simulink model "atrias_original"  (R2017a)
settings: Solver=ode45  StartTime=0.0  StopTime=sim_t  RelTol=1e-6  EnableMultiTasking=on
values from neighbouring files (symbols this model uses):
  N = grid_slice*1000    [createGrid.m]
  nm = fn_set_vnmc_params(sm, sample_time)    [kernel_scores_NM_mismatch.m]    (also in main_ATRIAS_cluster.m)
  nmc_BLCtrlPar = nmc.BLCtrlPar    [kernel_scores_NM_mismatch.m]    (also in main_ATRIAS_cluster.m)
  nmc_FPCtrlPar = nmc.FPCtrlPar    [kernel_scores_NM_mismatch.m]    (also in main_ATRIAS_cluster.m)
  nmc_LLCtrlPar = nmc.LLCtrlPar    [kernel_scores_NM_mismatch.m]    (also in main_ATRIAS_cluster.m)
  nmc_StCtrlPar = nmc.StCtrlPar    [kernel_scores_NM_mismatch.m]    (also in main_ATRIAS_cluster.m)
  nmc_SwCtrlPar = nmc.SwCtrlPar    [kernel_scores_NM_mismatch.m]    (also in main_ATRIAS_cluster.m)
  nmc_TrCtrlPar = nmc.TrCtrlPar    [kernel_scores_NM_mismatch.m]    (also in main_ATRIAS_cluster.m)
  nStep_switchCtrl = 10    [main_ATRIAS_cluster.m]
  nStep_thr = 1000    [createSimInitial.m]    (also in main_ATRIAS_cluster.m)
  rc_CtrlPar = [rc.k_placement, rc.T_step, rc.Cd, rc.kpt, rc.kdt, rc.desired_theta, rc.desired_z, rc.kpz, rc.kdz]    [kernel_scores_NM_mismatch.m]    (also in main_ATRIAS_cluster.m)
  sm = fn_set_MechParams(sm)    [kernel_scores_NM_mismatch.m]    (also in main_ATRIAS_cluster.m = fn_set_MechParams(sm,perturb))
  test_VNMC = 1    [createSimInitial.m]    (also in main_ATRIAS_cluster.m = 0)
undefined symbols (not defined in the file or in its folder): delta_phi_max, delta_phi_max_buffer, delta_phi_min, DiscIntNeverNeededParam, Discrete, idc, initial_dx_estimate, initial_dy_estimate, initial_dz_estimate, initial_z_estimate, kd_shin_max, kd_shin_min, kd_splay_max, kd_splay_min, kd_thigh_max, kd_thigh_min, kp_shin_max, kp_shin_min, kp_splay_max, kp_splay_min, kp_thigh_max, kp_thigh_min, mc, min_splay_angle, min_splay_buffer, phi_shin_max, phi_shin_max_buffer, phi_shin_min, phi_shin_min_buffer, phi_thigh_max, phi_thigh_max_buffer, phi_thigh_min, phi_thigh_min_buffer, rad, rc, s, sample_time, sgn, sim_d, t_friction, Time, X, Y, Z
libraries: sm_lib x202, nesl_utility x122, simulink x77, simulink_extras x24, fl_lib x16, mblibv1 x4, ctrlSharedLib x4, commnoisgen2 x1, dspswit3 x1
(part 1 of 17)
settings Model: TunableVars=nmc_BLCtrlPar,nmc_FPCtrlPar,nmc_LLCtrlPar,nmc_StCtrlPar,nmc_SwCtrlPar,nmc_TrCtrlPar  TunableVarsStorageClass=Auto,Auto,Auto,Auto,Auto,Auto  TunableVarsTypeQualifier=,,,,,  Creator=smsong  LastModifiedBy=arai
settings DataIOCC: InitialState=SimInitial  LimitDataPoints=on  SaveFinalState=on  SaveCompleteFinalSimState=on  SaveFormat=Array
settings OptimizationCC: EfficientMapNaN2IntZero=off  LifeSpan=inf
settings DebuggingCC: SFUnexpectedBacktrackingDiag=warning  SFNoUnconditionalDefaultTransitionDiag=warning  SFExecutionAtInitializationDiag=none
settings HardwareCC: ProdBitPerPointer=32  ProdBitPerSizeT=32  ProdBitPerPtrDiffT=32  ProdLargestAtomicFloat=None  ProdIntDivRoundTo=Undefined  ProdEndianess=Unspecified  ProdWordSize=32  ProdHWDeviceType=32-bit Generic  TargetBitPerLong=64  TargetBitPerPointer=64  TargetBitPerSizeT=64  TargetBitPerPtrDiffT=64  TargetLongLongMode=on  TargetIntDivRoundTo=Zero  TargetEndianess=LittleEndian  TargetWordSize=64  TargetHWDeviceType=MATLAB Host  ProdEqTarget=off
settings ModelReferenceCC: PropagateSignalLabelsOutOfModel=off
settings CodeAppCC: MaxIdLength=128
settings GRTTargetCC: TargetLangStandard=C89/C90 (ANSI)  CombineOutputUpdateFcns=off  GRTInterface=on  UseToolchainInfoCompliant=off
settings ConfigComp: CovMetricSettings=dw  CovHtmlReporting=on  CovSaveCumulativeToWorkspaceVar=on  CovSaveSingleToWorkspaceVar=on  CovExternalEMLEnable=off
settings ConfigurationSet: Description=SimMechanics 2G
settings ExplorerConfigSet: InternalSimMechanicsExplorerSettings="<ExplorerConfiguration><canonicalview>default</canonicalview><AnimationSetting><BasePlaybackSpeed>1.0</BasePlaybackSpeed><PlaybackSpeedFactor>1.0</PlaybackSpeedFactor></AnimationSetting><TilePanel><TileInfo><Tiles Columns=\"1\" Count=\"1\" Rows=\"1\"><Column Left=\"2\" Weight=\"1\"/><Column Left=\"738\"/><Row Top=\"2\" Weight=\"1\"/><Row Top=\"586\"/><Tile Height=\"1\" Width=\"1\" X=\"0\" Y=\"0\"/></Tiles></TileInfo><SceneInfo><SceneViewer><BGColor><R>1</R><G>1</G><B>1</B></BGColor><Camera><DoPerspective>off</DoPerspective><Position><X>-1.70399005576821305</X><Y>-4.20466739695413683</Y><Z>2.0578773047124157</Z></Position><Center><X>-0.00120101730655930439</X><Y>-0.00299649565581994182</Y><Z>1.48292546750794929</Z></Center><Up><X>0.0468067459368392558</X><Y>0.116782400880656612</Y><Z>0.992053929672855328</Z></Up><ViewLimDist>1</ViewLimDist><YLim>2.524026181051787</YLim><XLim>3.1912470149993899</XLim></Camera></SceneViewer></SceneInfo></TilePanel><MechEditorPanel><Cameras/><GfxPanelCameraMap/><VideoCreator><PlaybackSpeedRatio>1.0</PlaybackSpeedRatio><FrameRate>30</FrameRate><VideoFormat>Motion JPEG AVI</VideoFormat><FrameSize>auto</FrameSize></VideoCreator></MechEditorPanel></ExplorerConfiguration>"

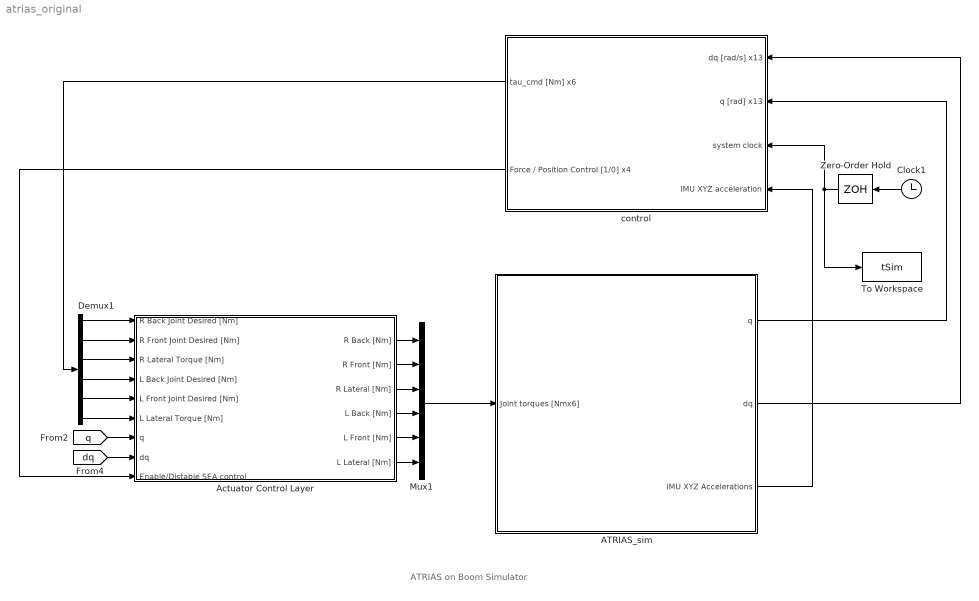
== system atrias_original ==
  note: ATRIAS on Boom Simulator
  ATRIAS_sim : Subsystem
  Actuator Control Layer : Subsystem
  Clock1 : Clock
  Demux1 : Demux  Outputs=6
  Mux1 : Mux  Inputs=6
  To Workspace : ToWorkspace  VariableName=tSim  SaveFormat=Timeseries  SampleTime=-1
      settings: MaxDataPoints=1
  Zero-Order Hold : ZeroOrderHold  SampleTime=sample_time
  control : Subsystem
  wires:
  Clock1/1 -> Zero-Order Hold/1
  Zero-Order Hold/1 -> To Workspace/1, control/3(system clock)
  [q] -> Actuator Control Layer/7(q)
  [dq] -> Actuator Control Layer/8(dq)
  Demux1/1 -> Actuator Control Layer/1(R Back Joint Desired [Nm])
  Demux1/2 -> Actuator Control Layer/2(R Front Joint Desired [Nm])
  Demux1/4 -> Actuator Control Layer/4(L Back Joint Desired [Nm])
  Demux1/5 -> Actuator Control Layer/5(L Front Joint Desired [Nm])
  Demux1/3 -> Actuator Control Layer/3(R Lateral Torque [Nm])
  Demux1/6 -> Actuator Control Layer/6(L Lateral Torque [Nm])
  Actuator Control Layer/3(R Lateral [Nm]) -> Mux1/3
  Actuator Control Layer/1(R Back [Nm]) -> Mux1/1
  Actuator Control Layer/2(R Front [Nm]) -> Mux1/2
  Actuator Control Layer/4(L Back [Nm]) -> Mux1/4
  Actuator Control Layer/5(L Front [Nm]) -> Mux1/5
  Actuator Control Layer/6(L Lateral [Nm]) -> Mux1/6
  Mux1/1 -> ATRIAS_sim/1(Joint torques [Nmx6])
  control/1(tau_cmd [Nm] x6) -> Demux1/1
  control/2(Force / Position Control [1/0] x4) -> Actuator Control Layer/9(Enable/Distable SEA control)
  ATRIAS_sim/2(dq) -> control/1(dq [rad/s] x13)
  ATRIAS_sim/1(q) -> control/2(q [rad] x13)
  ATRIAS_sim/3(IMU XYZ Accelerations) -> control/4(IMU XYZ acceleration)

== system atrias_original/ATRIAS_sim ==
  Joint torques [Nmx6] : Inport
  Acceleration Measurement : Scope  NumInputPorts=3
  Delay : Delay  DelayLength=1  SampleTime=sample_time
  Demux : Demux  Outputs=6
  Demux2 : Demux  Outputs=3
  Discrete Derivative : Subsystem
  Discretize : ZeroOrderHold  SampleTime=sample_time
  Discretize1 : ZeroOrderHold  SampleTime=sample_time
  Discretize2 : ZeroOrderHold  SampleTime=sample_time
  Gaussian Noise Generator : commnoisgen2/Gaussian Noise Generator  m=0  d=sm.sensor_noise_variance  s=41  Ts=sample_time  frameBased=off  sampPerFrame=1  orient=off  outDataType=double
  Mechanical System Layer : Subsystem
  Mux : Mux  Inputs=13
  Sum : Sum  Inputs=|++
  q : Outport  InitialOutput=[0]
  dq : Outport  Port=2  InitialOutput=[0]
  IMU XYZ Accelerations : Outport  Port=3  InitialOutput=[0]
  wires:
  Mechanical System Layer/1(R Back Joint [rad]) -> Mux/1
  Mechanical System Layer/2(R Back Gear [rad]) -> Mux/2
  Mechanical System Layer/3(R Front Joint [rad]) -> Mux/3
  Mechanical System Layer/4(R Front Gear [rad]) -> Mux/4
  Mechanical System Layer/5(L Back Joint [rad]) -> Mux/5
  Mechanical System Layer/6(L Back Gear [rad]) -> Mux/6
  Mechanical System Layer/7(L Front Joint [rad]) -> Mux/7
  Mechanical System Layer/8(L Front Gear [rad]) -> Mux/8
  Mechanical System Layer/9(R Lateral [rad]) -> Mux/9
  Mechanical System Layer/10(L Lateral [rad]) -> Mux/10
  Mechanical System Layer/11(Torso Roll [rad]) -> Mux/11
  Mechanical System Layer/12(Torso Yaw [rad]) -> Mux/12
  Mechanical System Layer/13(Torso Pitch [rad]) -> Mux/13
  Demux/1 -> Mechanical System Layer/1(R Back Motor [Nm])
  Demux/2 -> Mechanical System Layer/2(R Front Motor [Nm])
  Demux/3 -> Mechanical System Layer/3(R Lat Motor [Nm])
  Demux/4 -> Mechanical System Layer/4(L Back Motor [Nm])
  Demux/5 -> Mechanical System Layer/5(L Front Motor [Nm])
  Demux/6 -> Mechanical System Layer/6(L Lat Motor [Nm])
  Discretize/1 -> Sum/1
  Gaussian Noise Generator/1 -> ?
  Delay/1 -> Demux/1
  Mux/1 -> Discretize/1
  Mechanical System Layer/14("IMU XYZ Acclerations [m/s^2] x3 ") -> Discretize1/1
  Sum/1 -> q/1, Discrete Derivative/1(q)
  Joint torques [Nmx6]/1 -> Delay/1
  Discrete Derivative/1(dq) -> dq/1
  Demux2/3 -> Acceleration Measurement/3
  Demux2/1 -> Acceleration Measurement/1
  Demux2/2 -> Acceleration Measurement/2
  Discretize1/1 -> Demux2/1, Discretize2/1
  Discretize2/1 -> IMU XYZ Accelerations/1

== system atrias_original/Actuator Control Layer ==
  note: ATRIAS Actuation Control Layer
  note: q Order:
      |
      | backJointR
      | backGearR
      | frontJointR
      | frontGearR
      |
      | backJointL
      | backGearL
      | frontJointL
      | frontGearL
      |
      | latR
      | latL
      |
      | boomRoll
      | boomYaw
      | boomPitch
  R Back Joint Desired [Nm] : Inport
  R Front Joint Desired [Nm] : Inport  Port=2
  R Lateral Torque [Nm] : Inport  Port=3
  L Back Joint Desired [Nm] : Inport  Port=4
  L Front Joint Desired [Nm] : Inport  Port=5
  L Lateral Torque [Nm] : Inport  Port=6
  q : Inport  Port=7
  dq : Inport  Port=8
  Enable/Distable SEA control : Inport  Port=9
  Demux : Demux
  Gain : Gain  Gain=1/sm.mu_hmotor
  Gain1 : Gain  Gain=1/sm.mu_hmotor
  Mux : Mux
  Mux{3,5..7} (4 alike) : Mux  Inputs=2
  Product : Product
  "RB, RF, LB, LF" : Scope  NumInputPorts=4
  SEA Controller (Torque) : Subsystem
  Selector1 : Selector  InputPortWidth=13  IndexOptions=Index vector (dialog)  Indices=[2 4 6 8]  OutputSizes=1
  Selector10 : Selector  InputPortWidth=4  IndexOptions=Index vector (dialog)  Indices=[4]  OutputSizes=1
  Selector11 : Selector  InputPortWidth=4  IndexOptions=Index vector (dialog)  Indices=[2]  OutputSizes=1
  Selector12 : Selector  InputPortWidth=4  IndexOptions=Index vector (dialog)  Indices=[2]  OutputSizes=1
  Selector13 : Selector  InputPortWidth=4  IndexOptions=Index vector (dialog)  Indices=[1]  OutputSizes=1
  Selector14 : Selector  InputPortWidth=4  IndexOptions=Index vector (dialog)  Indices=[1]  OutputSizes=1
  Selector15 : Selector  InputPortWidth=13  IndexOptions=Index vector (dialog)  Indices=[1 3 5 7]  OutputSizes=1
  Selector16 : Selector  InputPortWidth=13  IndexOptions=Index vector (dialog)  Indices=[1 3 5 7]  OutputSizes=1
  Selector2 : Selector  InputPortWidth=13  IndexOptions=Index vector (dialog)  Indices=[2 4 6 8]  OutputSizes=1
  Selector7 : Selector  InputPortWidth=4  IndexOptions=Index vector (dialog)  Indices=[3]  OutputSizes=1
  Selector8 : Selector  InputPortWidth=4  IndexOptions=Index vector (dialog)  Indices=[3]  OutputSizes=1
  Selector9 : Selector  InputPortWidth=4  IndexOptions=Index vector (dialog)  Indices=[4]  OutputSizes=1
  Toggle SEA control : Subsystem
  tau_cmd [Nm] : Scope
  torque_command : ToWorkspace  VariableName=tau_cmd1  SampleTime=-1
  R Back [Nm] : Outport  InitialOutput=[0]
  R Front [Nm] : Outport  Port=2  InitialOutput=[0]
  R Lateral [Nm] : Outport  Port=3  InitialOutput=[0]
  L Back [Nm] : Outport  Port=4  InitialOutput=[0]
  L Front [Nm] : Outport  Port=5  InitialOutput=[0]
  L Lateral [Nm] : Outport  Port=6  InitialOutput=[0]
  wires:
  L Lateral Torque [Nm]/1 -> Gain1/1
  R Lateral Torque [Nm]/1 -> Gain/1
  Enable/Distable SEA control/1 -> SEA Controller (Torque)/6(Enable/Disable [1/0] x4), Product/2, Toggle SEA control/3(SEA Control on or off [1/0] x4)
  SEA Controller (Torque)/2(tau_cmd sagittal [Nm] x4) -> torque_command/1, Toggle SEA control/1(SEA Control Torques [Nm] x4)
  Product/1 -> Selector13/1, Selector9/1, Selector7/1, Selector11/1
  Demux/3 -> L Back [Nm]/1
  Demux/4 -> L Front [Nm]/1
  R Back Joint Desired [Nm]/1 -> Mux/1
  R Front Joint Desired [Nm]/1 -> Mux/2
  L Back Joint Desired [Nm]/1 -> Mux/3
  L Front Joint Desired [Nm]/1 -> Mux/4
  Selector15/1 -> SEA Controller (Torque)/2(phi_load [rad] x4)
  Selector2/1 -> SEA Controller (Torque)/3(phi_gear [rad] x4)
  Selector1/1 -> SEA Controller (Torque)/5(dphi_gear [rad/s] x4)
  Mux3/1 -> "RB, RF, LB, LF"/3
  Selector7/1 -> Mux3/1
  Selector8/1 -> Mux3/2
  Mux5/1 -> "RB, RF, LB, LF"/4
  Selector9/1 -> Mux5/1
  Selector10/1 -> Mux5/2
  Mux6/1 -> "RB, RF, LB, LF"/2
  Selector11/1 -> Mux6/1
  Selector12/1 -> Mux6/2
  Mux7/1 -> "RB, RF, LB, LF"/1
  SEA Controller (Torque)/1(tau_measured sagittal [Nm] x4) -> Selector14/1, Selector12/1, Selector8/1, Selector10/1
  Selector14/1 -> Mux7/2
  [dq] -> Selector16/1, Selector1/1
  Selector16/1 -> SEA Controller (Torque)/4(dphi_load [rad/s] x4)
  [q] -> Selector2/1, Selector15/1
  q/1 -> [q]
  dq/1 -> [dq]
  Demux/2 -> R Front [Nm]/1
  Demux/1 -> R Back [Nm]/1
  Selector13/1 -> Mux7/1
  Toggle SEA control/1(Motor Torque Commands [Nm] x4) -> tau_cmd [Nm]/1, Demux/1
  Mux/1 -> SEA Controller (Torque)/1(tau_des sagittal [Nm] x4), Toggle SEA control/2(Non-SEA control Torques [Nm] x4), Product/1
  Gain/1 -> R Lateral [Nm]/1
  Gain1/1 -> L Lateral [Nm]/1

== system atrias_original/control ==
  note: Robot-NMM Interface
  note: Neuromuscular Model
  note: Data
  note: Raibert Control
  note: Switch
  dq [rad/s] x13 : Inport
  q [rad] x13 : Inport  Port=2
  system clock : Inport  Port=3
  IMU XYZ acceleration : Inport  Port=4
  Data : Subsystem
  Demux3 : Demux
  Demux4 : Demux  Outputs=6
  Mux{,1,3..4} (4 alike) : Mux  Inputs=2
  Mux2 : Mux  Inputs=6
  Mux7 : Mux
  Mux8 : Mux
  NMM vs Raibert : Scope  NumInputPorts=4
  RC control : Subsystem
  Robot-to-NMM Interface : Subsystem
  Virtual Neuromuscular Control : Subsystem  SystemSampleTime=sample_time
  switch Ctrl : Subsystem
  tau_cmd [Nm] x6 : Outport
  Force / Position Control [1/0] x4 : Outport  Port=2  OutputWhenDisabled=reset  InitialOutput=[0 0 0 0 0 0]
  tag scope: LFootCnt=global, LLLoad=global, LLat_ctrl_trq=global, LLength=global, Lalpha=global, LdLength=global, Ldalpha=global, Ldgamma=global, Lgamma=global, Lphi12=global, Lphi23=global, Lshin_ctrl_trq=global, Lshin_ctrl_trq_NMM=global, Lshin_ctrl_trq_VMC=global, LtauB=global, LtauF=global, Lthigh_ctrl_trq=global, Lthigh_ctrl_trq_NMM=global, Lthigh_ctrl_trq_VMC=global, RFootCnt=global, RLLoad=global, RLat_ctrl_trq=global, RLength=global, Ralpha=global, RdLength=global, Rdalpha=global, Rdgamma=global, Rgamma=global, Rphi12=global, Rphi23=global, Rshin_ctrl_trq=global, Rshin_ctrl_trq_NMM=global, Rshin_ctrl_trq_VMC=global, RtauB=global, RtauF=global, Rthigh_ctrl_trq=global, Rthigh_ctrl_trq_NMM=global, Rthigh_ctrl_trq_VMC=global, dq=global, k_L=global, k_R=global, q=global
  wires:
  [Rshin_ctrl_trq] -> Mux2/1
  [Rthigh_ctrl_trq] -> Mux2/2
  [RLat_ctrl_trq] -> Mux2/3
  [Lshin_ctrl_trq] -> Mux2/4
  [Lthigh_ctrl_trq] -> Mux2/5
  [LLat_ctrl_trq] -> Mux2/6
  dq [rad/s] x13/1 -> [dq]
  q [rad] x13/1 -> [q]
  [q] -> Robot-to-NMM Interface/1(q_discrete [rad] x13)
  [dq] -> Robot-to-NMM Interface/2(dq_discrete [rad/2] x13)
  Robot-to-NMM Interface/23(L Leg Load [bw]) -> [LLLoad]
  Robot-to-NMM Interface/24(R Leg Load [bw]) -> [RLLoad]
  Robot-to-NMM Interface/6(L Alpha [rad]) -> [Lalpha]
  Robot-to-NMM Interface/5(R Alpha [rad]) -> [Ralpha]
  Robot-to-NMM Interface/8(L Leg Length [m]) -> [LLength]
  Robot-to-NMM Interface/7(R Leg Length [m]) -> [RLength]
  Robot-to-NMM Interface/4(L_tau_front_meas [Nm]) -> [LtauF]
  Robot-to-NMM Interface/3(L_tau_back_meas [Nm]) -> [LtauB]
  Robot-to-NMM Interface/2(R_tau_front_meas [Nm]) -> [RtauF]
  Robot-to-NMM Interface/1(R_tau_back_meas [Nm]) -> [RtauB]
  Robot-to-NMM Interface/11(R virtual knee angle [rad]) -> [Rphi12]
  Robot-to-NMM Interface/12(R virtual hip angle [rad]) -> [Rphi23]
  Robot-to-NMM Interface/13(L virtual knee angle [rad]) -> [Lphi12]
  Robot-to-NMM Interface/14(L virtual hip angle [rad]) -> [Lphi23]
  Robot-to-NMM Interface/16(L Jacobian Constant (k)) -> [k_L]
  Robot-to-NMM Interface/15(R Jacobian Constant (k)) -> [k_R]
  Robot-to-NMM Interface/21(R dAlpha [rad/s]) -> [Rdalpha]
  Robot-to-NMM Interface/22(L dAlpha [rad/s]) -> [Ldalpha]
  Robot-to-NMM Interface/17(Rgamma [rad]) -> [Rgamma]
  Robot-to-NMM Interface/18(Lgamma [rad]) -> [Lgamma]
  Robot-to-NMM Interface/19(Rdgamma [rad]) -> [Rdgamma]
  Robot-to-NMM Interface/20(Ldgamma [rad]) -> [Ldgamma]
  Robot-to-NMM Interface/10(R Leg Length Velocity [m/s]) -> [RdLength]
  Robot-to-NMM Interface/9(L Leg Length Velocity [m/s]) -> [LdLength]
  Demux4/1 -> [Rshin_ctrl_trq_VMC]
  Demux4/2 -> [Rthigh_ctrl_trq_VMC]
  Demux4/3 -> [RLat_ctrl_trq]
  Demux4/4 -> [Lshin_ctrl_trq_VMC]
  Virtual Neuromuscular Control/1(RtauB_des [Nm]) -> [Rshin_ctrl_trq_NMM]
  Virtual Neuromuscular Control/2(RtauF_des [Nm]) -> [Rthigh_ctrl_trq_NMM]
  Virtual Neuromuscular Control/3(LtauB_des [Nm]) -> [Lshin_ctrl_trq_NMM]
  Virtual Neuromuscular Control/4(LtauF_des [Nm]) -> [Lthigh_ctrl_trq_NMM]
  [Rshin_ctrl_trq_NMM] -> Mux/1, Mux7/1
  [Rthigh_ctrl_trq_NMM] -> Mux1/1, Mux7/2
  [Lshin_ctrl_trq_NMM] -> Mux3/1, Mux7/3
  [Lthigh_ctrl_trq_NMM] -> Mux4/1, Mux7/4
  [Rshin_ctrl_trq_VMC] -> Mux/2, Mux8/1
  [Rthigh_ctrl_trq_VMC] -> Mux1/2, Mux8/2
  [Lshin_ctrl_trq_VMC] -> Mux3/2, Mux8/3
  [Lthigh_ctrl_trq_VMC] -> Mux4/2, Mux8/4
  Demux3/4 -> [Lthigh_ctrl_trq]
  Demux3/3 -> [Lshin_ctrl_trq]
  Demux3/2 -> [Rthigh_ctrl_trq]
  Demux3/1 -> [Rshin_ctrl_trq]
  Robot-to-NMM Interface/26(L Contact [0/1]) -> [LFootCnt]
  Robot-to-NMM Interface/25(R Contact [0/1]) -> [RFootCnt]
  [dq] -> RC control/2(dq_cmu)
  [q] -> RC control/1(q_cmu)
  system clock/1 -> RC control/3(system clock)
  RC control/2(Motor Torque Command [Nm] x6) -> Demux4/1
  Demux4/5 -> [Lthigh_ctrl_trq_VMC]
  Demux4/6 -> [LLat_ctrl_trq]
  RC control/1(Force / Position Control [1/0] x4) -> Force / Position Control [1/0] x4/1
  Robot-to-NMM Interface/27(Entering stance) -> RC control/4(Entering Stance)
  IMU XYZ acceleration/1 -> RC control/5(Body XYZ Acceleration [m/s^2] x3)
  Mux/1 -> NMM vs Raibert/1
  Mux1/1 -> NMM vs Raibert/2
  Mux3/1 -> NMM vs Raibert/3
  Mux4/1 -> NMM vs Raibert/4
  switch Ctrl/1(selected) -> Demux3/1
  Mux7/1 -> switch Ctrl/1(VNMC)
  Mux8/1 -> switch Ctrl/2(RC)
  Mux2/1 -> tau_cmd [Nm] x6/1

== system atrias_original/ATRIAS_sim/Discrete Derivative ==
  q : Inport
  Gain1 : Gain  Gain=1/sample_time
  discrete difference : Subsystem
  dq : Outport
  wires:
  q/1 -> discrete difference/1(in)
  Gain1/1 -> dq/1
  discrete difference/1(out) -> Gain1/1

== system atrias_original/ATRIAS_sim/Mechanical System Layer ==
  R Back Motor [Nm] : Inport
  R Front Motor [Nm] : Inport  Port=2
  R Lat Motor [Nm] : Inport  Port=3
  L Back Motor [Nm] : Inport  Port=4
  L Front Motor [Nm] : Inport  Port=5
  L Lat Motor [Nm] : Inport  Port=6
  Boom : Subsystem
      mask Display: image('../images/boom.png');
  Boom Base : Subsystem
      mask Display: image('../images/boom_base.png');
  Demux : Demux  Outputs=3
  Demux1 : Demux  Outputs=3
  Demux2 : Demux  Outputs=3
  Floor : Subsystem
  Floor Frame : sm_lib/Frames and Transforms/Rigid Transform  TranslationMethod=Cartesian  TranslationStandardOffset=0  TranslationLengthUnit=m  TranslationStandardAxis=+Z  TranslationCartesianOffset=[0 -0.03 0]  TranslationROffset=0  TranslationROffsetUnits=m  TranslationZOffset=0  TranslationZOffsetUnits=m  TranslationThetaOffset=0  TranslationThetaOffsetUnits=deg  RotationMethod=AlignedAxes  RotationAngleUnits=deg  RotationStandardAxis=+Z  RotationAngle=0  RotationArbitraryAxis=[0 0 1]  FollAlignAxisA=+Z  BaseAlignAxisA=+Y  FollAlignAxisB=+X  BaseAlignAxisB=+X  RotationSequenceAxes=FollowerAxes  RotationSequence=XYX  RotationSequenceAngles=[0 0 0]  RotationSequenceAnglesUnits=deg  RotationMatrix=[1 0 0; 0 1 0; 0 0 1]
  From1 : From  Commented=on  GotoTag=GlobalRightLeftPrimary  TagVisibility=global
  From55 : From  Commented=on  GotoTag=RightLeftPrimary
  Gain : Gain  Commented=on  Gain=[1 -1 1]
  Goto : Goto  Commented=on  GotoTag=GlobalPrimaryGRF  TagVisibility=global
  Ground : Subsystem
  Ground Height : Scope  Commented=on
  L GRF : Scope
  L Ground Contact : Subsystem  SystemSampleTime=t_friction
  L Hip Shaft : Subsystem
      mask Display: image(flipdim(imread('../images/hipshaft.JPG'),2));
  L Leg : Subsystem
      mask Display: image('../images/leg.JPG');
  Left Hip Roll Joint : Subsystem
  Pitch Joint : Subsystem
  R GRF : Scope
  R Ground Contact : Subsystem  SystemSampleTime=t_friction
  R Hip Shaft : Subsystem
      mask Display: image('../images/hipshaft.JPG');
  R Leg : Subsystem
      mask Display: image('../images/leg.JPG');
  Right Hip Roll Joint : Subsystem
  Selector : Selector  Commented=on  InputPortWidth=3  IndexOptions=Index vector (dialog)  Indices=[1 3 2]  OutputSizes=1
  Sum : Sum  Inputs=2
  Switch : Switch  Commented=on  Criteria=u2 ~= 0
  Switch1 : Switch  Commented=on  Criteria=u2 ~= 0
  Terminator : Terminator
  Terminator1 : Terminator
  Terminator2 : Terminator
  Torso : Subsystem
      mask Display: image('../images/torso.png');
  Winch : Subsystem
  World to Yup : sm_lib/Frames and Transforms/Rigid Transform  TranslationMethod=None  TranslationStandardOffset=0  TranslationLengthUnit=m  TranslationStandardAxis=+Z  TranslationCartesianOffset=0  TranslationROffset=0  TranslationROffsetUnits=m  TranslationZOffset=0  TranslationZOffsetUnits=m  TranslationThetaOffset=0  TranslationThetaOffsetUnits=deg  RotationMethod=AlignedAxes  RotationAngleUnits=deg  RotationStandardAxis=+Z  RotationAngle=0  RotationArbitraryAxis=[0 0 1]  FollAlignAxisA=+Y  BaseAlignAxisA=+Z  FollAlignAxisB=+X  BaseAlignAxisB=+X  RotationSequenceAxes=FollowerAxes  RotationSequence=XYX  RotationSequenceAngles=[0 0 0]  RotationSequenceAnglesUnits=deg  RotationMatrix=[1 0 0; 0 1 0; 0 0 1]
  Yaw Joint : Subsystem
  Yaw Shaft : Subsystem
      mask Display: image('../images/boom_yaw_shaft.png');
  R Back Joint [rad] : Outport
  R Back Gear [rad] : Outport  Port=2
  R Front Joint [rad] : Outport  Port=3
  R Front Gear [rad] : Outport  Port=4
  L Back Joint [rad] : Outport  Port=5
  L Back Gear [rad] : Outport  Port=6
  L Front Joint [rad] : Outport  Port=7
  L Front Gear [rad] : Outport  Port=8
  R Lateral [rad] : Outport  Port=9
  L Lateral [rad] : Outport  Port=10
  Torso Roll [rad] : Outport  Port=11
  Torso Yaw [rad] : Outport  Port=12
  Torso Pitch [rad] : Outport  Port=13
  "IMU XYZ Acclerations [m/s^2] x3 " : Outport  Port=14
  tag scope: GRFz=global
  wires:
  L Leg/1(Shin Joint [rad]) -> L Back Joint [rad]/1
  R Back Motor [Nm]/1 -> R Leg/1(Shin Motor [Nm])
  L Back Motor [Nm]/1 -> L Leg/1(Shin Motor [Nm])
  Right Hip Roll Joint/1(Hip Roll [rad]) -> R Lateral [rad]/1
  L Leg/3(Thigh Joint [rad]) -> L Front Joint [rad]/1
  Left Hip Roll Joint/1(Hip Roll [rad]) -> L Lateral [rad]/1
  L Leg/4(Thigh Gear [rad]) -> L Front Gear [rad]/1
  R Leg/1(Shin Joint [rad]) -> R Back Joint [rad]/1
  R Leg/2(Shin Gear [rad]) -> R Back Gear [rad]/1
  L Leg/2(Shin Gear [rad]) -> L Back Gear [rad]/1
  R Leg/4(Thigh Gear [rad]) -> R Front Gear [rad]/1
  L Front Motor [Nm]/1 -> L Leg/2("Thigh Motor [Nm]  ")
  R Lat Motor [Nm]/1 -> Right Hip Roll Joint/1(Hip Motor [Nm])
  R Front Motor [Nm]/1 -> R Leg/2("Thigh Motor [Nm]  ")
  L Lat Motor [Nm]/1 -> Left Hip Roll Joint/1(Hip Motor [Nm])
  R Leg/3(Thigh Joint [rad]) -> R Front Joint [rad]/1
  Pitch Joint/1(Pitch [rad]) -> Terminator/1
  Yaw Joint/1(Yaw [rad]) -> Terminator1/1
  From55/1 -> Switch/2
  Switch/1 -> Ground Height/1
  L Ground Contact/2(zGround) -> Switch/3
  R Ground Contact/2(zGround) -> Switch/1
  Torso/1(IMU XYZ Accelerations [m/s^2] x3) -> "IMU XYZ Acclerations [m/s^2] x3 "/1
  Torso/2(IMU Orientation [rad x3]) -> Demux/1
  Demux/1 -> Torso Roll [rad]/1
  Demux/2 -> Torso Pitch [rad]/1
  Winch/1(Boom Roll [rad]) -> Terminator2/1
  Demux/3 -> Torso Yaw [rad]/1
  From1/1 -> Switch1/2
  L Ground Contact/1(GRF) -> Demux1/1, Switch1/3, L GRF/1
  R Ground Contact/1(GRF) -> Demux2/1, Switch1/1, R GRF/1
  Switch1/1 -> Selector/1
  Selector/1 -> Gain/1
  Gain/1 -> Goto/1
  Demux1/3 -> Sum/1
  Demux2/3 -> Sum/2
  Sum/1 -> [GRFz]
  connections:
  Torso/LConn1 -- Left Hip Roll Joint/RConn1
  Right Hip Roll Joint/RConn1 -- R Hip Shaft/RConn1
  Winch/RConn2 -- Yaw Shaft/RConn1
  Left Hip Roll Joint/LConn1 -- L Hip Shaft/LConn1
  R Ground Contact/LConn1 -- R Leg/LConn1
  R Leg/RConn1 -- R Hip Shaft/LConn1
  Torso/LConn2 -- Right Hip Roll Joint/LConn1
  L Ground Contact/LConn1 -- L Leg/RConn1
  Pitch Joint/LConn1 -- Torso/RConn1
  Floor Frame/RConn1 -- Floor/LConn1
  World to Yup/LConn1 -- Ground/RConn1
  Boom/LConn1 -- Winch/RConn1
  Yaw Shaft/LConn1 -- Yaw Joint/RConn1
  Yaw Joint/LConn1 -- Boom Base/RConn1
  Pitch Joint/RConn1 -- Boom/RConn1
  L Hip Shaft/RConn1 -- L Leg/LConn1
  Floor Frame/LConn1 -- World to Yup/RConn1 -- Boom Base/LConn1

== system atrias_original/Actuator Control Layer/SEA Controller (Torque) ==
  tau_des sagittal [Nm] x4 : Inport
  phi_load [rad] x4 : Inport  Port=2
  phi_gear [rad] x4 : Inport  Port=3
  dphi_load [rad/s] x4 : Inport  Port=4
  dphi_gear [rad/s] x4 : Inport  Port=5
  Enable/Disable [1/0] x4 : Inport  Port=6
  Desired Torque Derivative : Subsystem
  Detect Change : simulink/Logic and Bit Operations/Detect Change  vinit=0  InputProcessing=Inherited  OutDataTypeStr=boolean
  Spring Stiffness1 : Gain  Gain=mc.k_leg_spring
  Spring Stiffness2 : Gain  Gain=mc.k_leg_spring
  Sum10 : Sum  Inputs=-+|
  Sum11 : Sum  Inputs=|++
  Sum6 : Sum  Inputs=-+|
  Sum7 : Sum  Inputs=|+-
  Sum8 : Sum  Inputs=+++
  Sum9 : Sum  Inputs=|+-
  Torque Limiter (outside) 1 : Saturate  UpperLimit=sm.LEG_MTR_MAX_TORQUE  LowerLimit=-sm.LEG_MTR_MAX_TORQUE  ZeroCross=off
      settings: AttributesFormatString=Hi: %<UpperLimit>\nLo: %<LowerLimit>
  kd_gain : Gain  Description=xPCTag(1)=kd_sea_torque;  Gain=mc.kd_sea_torque
  kd_gain2 : Gain  Description=xPCTag(1)=kd_sea_torque;  Gain=mc.kp_sea_torque
  tau_measured sagittal [Nm] x4 : Outport
  tau_cmd sagittal [Nm] x4 : Outport  Port=2
  wires:
  Sum9/1 -> kd_gain2/1
  Torque Limiter (outside) 1/1 -> tau_cmd sagittal [Nm] x4/1
  kd_gain2/1 -> Sum11/1
  kd_gain/1 -> Sum11/2
  Sum11/1 -> Sum8/2
  Sum6/1 -> Spring Stiffness1/1
  Sum8/1 -> Torque Limiter (outside) 1/1
  Sum7/1 -> kd_gain/1
  dphi_gear [rad/s] x4/1 -> Sum10/2
  dphi_load [rad/s] x4/1 -> Sum10/1
  Spring Stiffness2/1 -> Sum7/2
  Sum10/1 -> Spring Stiffness2/1
  Desired Torque Derivative/1(Derivative x4) -> Sum7/1
  phi_gear [rad] x4/1 -> Sum6/2
  phi_load [rad] x4/1 -> Sum6/1
  Spring Stiffness1/1 -> tau_measured sagittal [Nm] x4/1, Sum9/2, Sum8/1
  Detect Change/1 -> Desired Torque Derivative/2(Reset [1/0] x4)
  tau_des sagittal [Nm] x4/1 -> Desired Torque Derivative/1(Signal x4), Sum9/1
  Enable/Disable [1/0] x4/1 -> Detect Change/1

== system atrias_original/Actuator Control Layer/Toggle SEA control ==
  SEA Control Torques [Nm] x4 : Inport
  Non-SEA control Torques [Nm] x4 : Inport  Port=2
  SEA Control on or off [1/0] x4 : Inport  Port=3
  Demux2 : Demux
  Demux3 : Demux
  Demux4 : Demux
  Mux1 : Mux
  Switch{,1..3} (4 alike) : Switch  Criteria=u2 > Threshold
  Motor Torque Commands [Nm] x4 : Outport
  wires:
  SEA Control Torques [Nm] x4/1 -> Demux4/1
  Demux2/3 -> Switch3/2
  Switch3/1 -> Mux1/3
  Demux4/4 -> Switch2/1
  Demux2/1 -> Switch1/2
  Demux4/3 -> Switch3/1
  Demux3/1 -> Switch1/3
  Demux2/2 -> Switch/2
  Demux3/3 -> Switch3/3
  Demux3/2 -> Switch/3
  Demux3/4 -> Switch2/3
  Switch2/1 -> Mux1/4
  Demux4/1 -> Switch1/1
  SEA Control on or off [1/0] x4/1 -> Demux2/1
  Demux4/2 -> Switch/1
  Non-SEA control Torques [Nm] x4/1 -> Demux3/1
  Demux2/4 -> Switch2/2
  Mux1/1 -> Motor Torque Commands [Nm] x4/1
  Switch/1 -> Mux1/2
  Switch1/1 -> Mux1/1

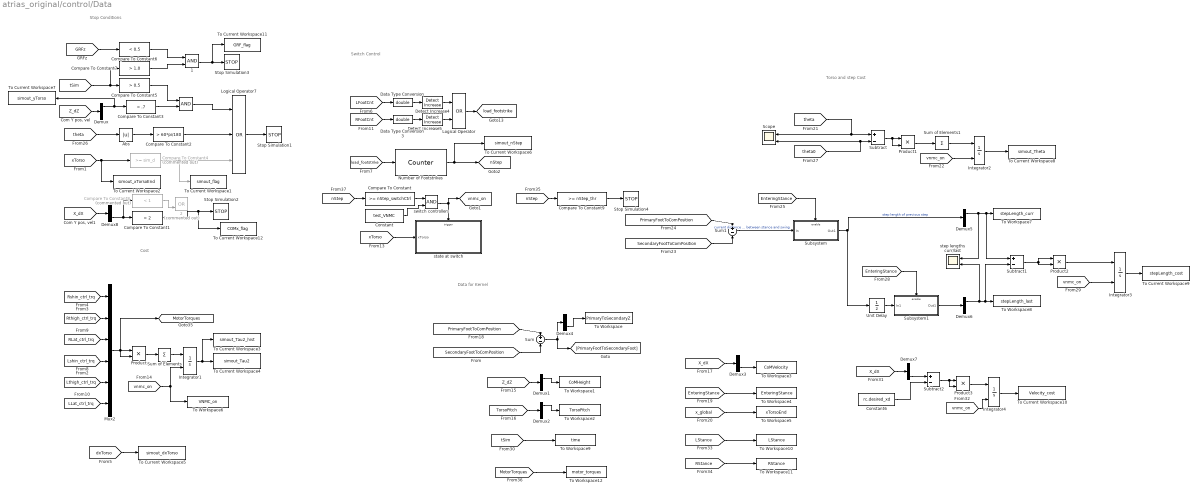
== system atrias_original/control/Data ==
  note: Stop Conditions
  note: Cost
  note: Switch Control
  note: Data for Kernel
  note: Torso and step Cost
  " " : Logic  AllPortsSameDT=off  OutDataTypeStr=boolean
  " 1" : Logic  AllPortsSameDT=off  OutDataTypeStr=boolean
  " 2" : Logic  Commented=on  Operator=OR  AllPortsSameDT=off  OutDataTypeStr=boolean
  Abs : Abs
  Compare To Constant : simulink/Logic and Bit Operations/Compare To Constant  relop=>=  const=nStep_switchCtrl  OutDataTypeStr=boolean
  Compare To Constant1 : simulink/Logic and Bit Operations/Compare To Constant  relop=>  const=2  OutDataTypeStr=boolean
  Compare To Constant2 : simulink/Logic and Bit Operations/Compare To Constant  relop=>  const=60*pi/180  OutDataTypeStr=boolean
  Compare To Constant3 : simulink/Logic and Bit Operations/Compare To Constant  relop=<  const=.7  OutDataTypeStr=boolean
  Compare To Constant4 : simulink/Logic and Bit Operations/Compare To Constant  Commented=on  relop=>=  const=sim_d  OutDataTypeStr=boolean
  Compare To Constant5 : simulink/Logic and Bit Operations/Compare To Constant  relop=>  const=0.5  OutDataTypeStr=boolean
  Compare To Constant6 : simulink/Logic and Bit Operations/Compare To Constant  relop=<  const=0.5  OutDataTypeStr=boolean  ZeroCross=off
  Compare To Constant7 : simulink/Logic and Bit Operations/Compare To Constant  relop=>  const=1.0  OutDataTypeStr=boolean  ZeroCross=off
  Compare To Constant8 : simulink/Logic and Bit Operations/Compare To Constant  Commented=on  relop=<  const=1  OutDataTypeStr=boolean
  Compare To Constant9 : simulink/Logic and Bit Operations/Compare To Constant  relop=>=  const=nStep_thr  OutDataTypeStr=boolean
  Constant : Constant  Value=test_VNMC
  Constant6 : Constant  Value=rc.desired_xd
  Data Type Conversion : DataTypeConversion  OutDataTypeStr=double
  Data Type Conversion3 : DataTypeConversion  OutDataTypeStr=double
  Demux{,1..3,7..8} (6 alike) : Demux  Outputs=2
  Demux4 : Demux  Outputs=3
  Demux5 : Demux  Outputs=3
  Demux6 : Demux  Outputs=3
  Detect Increase4 : simulink/Logic and Bit Operations/Detect Increase  vinit=0.0  InputProcessing=Inherited  OutDataTypeStr=boolean
  Detect Increase5 : simulink/Logic and Bit Operations/Detect Increase  vinit=0.0  InputProcessing=Inherited  OutDataTypeStr=boolean
  Integrator{1..4} (4 alike) : Integrator  ExternalReset=rising  ZeroCross=off
  Logical Operator : Logic  Operator=OR  AllPortsSameDT=off  OutDataTypeStr=boolean
  Logical Operator7 : Logic  Operator=OR  Inputs=3  AllPortsSameDT=off  OutDataTypeStr=boolean
  Mux2 : Mux  Inputs=6
  Number of Footstrikes : dspswit3/Counter  Direction=Up  CountEvent=Rising edge  CounterSize=User defined  MaxCount=255  InitialCount=0  Output=Count  HitValue=4  ResetInput=off  SamplesPerFrame=1  Ts=1  CntDtype=double  HitDtype=Boolean
  Product{,1..3} (4 alike) : Product
  Scope : Scope  NumInputPorts=2
  Stop Simulation{1..4} (4 alike) : Stop
  Subsystem : Subsystem
  Subsystem1 : Subsystem
  Subtract : Sum  Inputs=+-
  Subtract1 : Sum  Inputs=+-
  Subtract2 : Sum  Inputs=+-
  Sum : Sum  Inputs=+-
  Sum of Elements : Sum  Inputs=+
  Sum of Elements1 : Sum  Inputs=+
  Sum1 : Sum  Inputs=+-
  To Current Workspace1 : ToWorkspace  VariableName=simout_flag  SaveFormat=Structure  SampleTime=-1
      settings: MaxDataPoints=1
  To Current Workspace10 : ToWorkspace  VariableName=Velocity_cost  SaveFormat=Structure With Time  SampleTime=-1
  To Current Workspace11 : ToWorkspace  VariableName=GRF_flag  SaveFormat=Structure  SampleTime=-1
      settings: MaxDataPoints=1
  To Current Workspace12 : ToWorkspace  VariableName=COMx_flag  SaveFormat=Structure  SampleTime=-1
      settings: MaxDataPoints=1
  To Current Workspace2 : ToWorkspace  VariableName=simout_xTorsoEnd  SaveFormat=Structure With Time  SampleTime=-1
  To Current Workspace3 : ToWorkspace  VariableName=simout_Tau2_hist  SaveFormat=Structure With Time  SampleTime=-1
  To Current Workspace4 : ToWorkspace  VariableName=simout_Tau2  SaveFormat=Structure  SampleTime=-1
      settings: MaxDataPoints=1
  To Current Workspace5 : ToWorkspace  VariableName=simout_dxTorso  SaveFormat=Structure With Time  SampleTime=-1
  To Current Workspace6 : ToWorkspace  VariableName=simout_nStep  SaveFormat=Structure With Time  SampleTime=-1
  To Current Workspace7 : ToWorkspace  VariableName=simout_yTorso  SaveFormat=Structure With Time  SampleTime=-1
  To Current Workspace8 : ToWorkspace  VariableName=simout_Theta  SaveFormat=Structure With Time  SampleTime=-1
  To Current Workspace9 : ToWorkspace  VariableName=stepLength_cost  SaveFormat=Structure  SampleTime=-1
  To Workspace : ToWorkspace  VariableName=PrimaryToSecondaryZ  SaveFormat=Structure With Time  SampleTime=-1
  To Workspace1 : ToWorkspace  VariableName=CoMHeight  SaveFormat=Structure With Time  SampleTime=-1
  To Workspace10 : ToWorkspace  VariableName=LStance  SaveFormat=Structure With Time  SampleTime=-1
  To Workspace11 : ToWorkspace  VariableName=RStance  SaveFormat=Structure With Time  SampleTime=-1
  To Workspace12 : ToWorkspace  VariableName=motor_torques  SaveFormat=Structure With Time  SampleTime=-1
  To Workspace2 : ToWorkspace  VariableName=TorsoPitch  SaveFormat=Structure With Time  SampleTime=-1
  To Workspace3 : ToWorkspace  VariableName=CoMVelocity  SaveFormat=Structure With Time  SampleTime=-1
  To Workspace4 : ToWorkspace  VariableName=EnteringStance  SaveFormat=Structure With Time  SampleTime=-1
  To Workspace5 : ToWorkspace  VariableName=xTorsoEnd  SaveFormat=Structure With Time  SampleTime=-1
  To Workspace6 : ToWorkspace  VariableName=VNMC_on  SaveFormat=Structure With Time  SampleTime=-1
  To Workspace7 : ToWorkspace  VariableName=stepLength_curr  SaveFormat=Structure With Time  SampleTime=-1
  To Workspace8 : ToWorkspace  VariableName=stepLength_last  SaveFormat=Structure With Time  SampleTime=-1
  To Workspace9 : ToWorkspace  VariableName=time  SaveFormat=Structure With Time  SampleTime=-1
  Unit Delay : UnitDelay  SampleTime=-1
  state at switch : Subsystem  TreatAsAtomicUnit=on
  step lengths curr/last : Scope  NumInputPorts=2
  switch controllers : Logic  AllPortsSameDT=off  OutDataTypeStr=boolean
  tag scope: MotorTorques=global, load_footstrike=global, nStep=global, vnmc_on=global
  wires:
  Logical Operator7/1 -> Stop Simulation1/1
  [theta] -> Abs/1
  Abs/1 -> Compare To Constant2/1
  Compare To Constant2/1 -> Logical Operator7/2
  Compare To Constant4/1 -> Logical Operator7/3, To Current Workspace1/1
  [xTorso] -> Compare To Constant4/1, To Current Workspace2/1
  [Rshin_ctrl_trq] -> Mux2/1
  [Rthigh_ctrl_trq] -> Mux2/2
  [RLat_ctrl_trq] -> Mux2/3
  [Lshin_ctrl_trq] -> Mux2/4
  [Lthigh_ctrl_trq] -> Mux2/5
  [LLat_ctrl_trq] -> Mux2/6
  Sum of Elements/1 -> Integrator1/1
  Product/1 -> Sum of Elements/1
  Mux2/1 -> [MotorTorques], Product/2, Product/1
  Integrator1/1 -> To Current Workspace3/1, To Current Workspace4/1
  [load_footstrike] -> Number of Footstrikes/1
  Number of Footstrikes/1 -> To Current Workspace6/1, [nStep]
  [LFootCnt] -> Data Type Conversion/1
  [RFootCnt] -> Data Type Conversion3/1
  Detect Increase4/1 -> Logical Operator/1
  Detect Increase5/1 -> Logical Operator/2
  Logical Operator/1 -> [load_footstrike]
  Data Type Conversion/1 -> Detect Increase4/1
  Data Type Conversion3/1 -> Detect Increase5/1
  [dxTorso] -> To Current Workspace5/1
  [nStep] -> Compare To Constant/1
  switch controllers/1 -> [vnmc_on], state at switch/Trigger
  [xTorso] -> state at switch/1(xTorso)
  [vnmc_on] -> Integrator1/2, To Workspace6/1
  Compare To Constant3/1 -> " "/2
  [Z_dZ] -> Demux/1
  Demux/1 -> To Current Workspace7/1, Compare To Constant3/1
  [tSim] -> Compare To Constant7/1, Compare To Constant5/1
  Compare To Constant5/1 -> " "/1
  " "/1 -> Logical Operator7/1
  Sum/1 -> Demux4/1, [PrimaryFootToSecondaryFoot]
  [SecondaryFootToComPosition] -> Sum/2
  [PrimaryFootToComPosition] -> Sum/1
  [Z_dZ] -> Demux1/1
  Demux1/1 -> To Workspace1/1
  [TorsoPitch] -> Demux2/1
  Demux2/1 -> To Workspace2/1
  [X_dX] -> Demux3/1
  Demux3/2 -> To Workspace3/1
  Demux4/3 -> To Workspace/1
  [EnteringStance] -> To Workspace4/1
  [x_global] -> To Workspace5/1
  [theta0] -> Subtract/2, Scope/2
  Subtract/1 -> Product1/2, Product1/1
  [vnmc_on] -> Integrator2/2
  Integrator2/1 -> To Current Workspace8/1
  [SecondaryFootToComPosition] -> Sum1/2
  [PrimaryFootToComPosition] -> Sum1/1
  Demux5/1 -> step lengths curr/last/1, Subtract1/1, To Workspace7/1
  Sum1/1 -> Subsystem/1(In)  "current distance  between stance and swing"
  Demux6/1 -> step lengths curr/last/2, Subtract1/2, To Workspace8/1
  Subsystem/1(Out1) -> Unit Delay/1, Demux5/1  "step length of previous step"
  Subsystem1/1(Out1) -> Demux6/1
  Unit Delay/1 -> Subsystem1/1(In1)
  [EnteringStance] -> Subsystem/Enable
  [EnteringStance] -> Subsystem1/Enable
  Subtract1/1 -> Product2/1, Product2/2
  Product2/1 -> Integrator3/1
  [vnmc_on] -> Integrator3/2
  Integrator3/1 -> To Current Workspace9/1
  [tSim] -> To Workspace9/1
  Product1/1 -> Sum of Elements1/1
  Sum of Elements1/1 -> Integrator2/1
  [theta] -> Subtract/1, Scope/1
  [X_dX] -> Demux7/1
  Demux7/2 -> Subtract2/1
  Constant6/1 -> Subtract2/2
  Subtract2/1 -> Product3/2, Product3/1
  Product3/1 -> Integrator4/1
  [vnmc_on] -> Integrator4/2
  Integrator4/1 -> To Current Workspace10/1
  [X_dX] -> Demux8/1
  Demux8/2 -> Compare To Constant8/1, Compare To Constant1/1
  [GRFz] -> Compare To Constant6/1
  Compare To Constant6/1 -> " 1"/1
  " 1"/1 -> To Current Workspace11/1, Stop Simulation3/1
  Compare To Constant7/1 -> " 1"/2
  Compare To Constant1/1 -> To Current Workspace12/1, Stop Simulation2/1
  Compare To Constant8/1 -> " 2"/2
  [LStance] -> To Workspace10/1
  [RStance] -> To Workspace11/1
  [nStep] -> Compare To Constant9/1
  Compare To Constant9/1 -> Stop Simulation4/1
  [MotorTorques] -> To Workspace12/1
  Compare To Constant/1 -> switch controllers/1
  Constant/1 -> switch controllers/2
